simulink model "RelOrbSim"  (R2021b)
settings: Solver=ode3  StartTime=0.0  StopTime=600  FixedStep=1  MaxStep=0.1  RelTol=1e-13  AbsTol=1e-16
values from neighbouring files (symbols this model uses):
  ctrl_flag = 1    [MAIN.m]    (also in MAIN_TestCampaign_1.m)
  g0 = 9.81    [MAIN.m]    (also in MAIN_TestCampaign_1.m)
  Isp = 450    [MAIN.m]    (also in MAIN_TestCampaign_1.m)
  J2_flag = 0    [MAIN.m]    (also in MAIN_TestCampaign_1.m)
  M0 = 12    [MAIN.m]    (also in MAIN_TestCampaign_1.m)
  Mp = 0.5    [MAIN.m]    (also in MAIN_TestCampaign_1.m)
  Y0_Chaser = [7106.14, 0.501, deg2rad(98.31), deg2rad(0), deg2rad(270), deg2rad(0)]'    [MAIN.m]    (also in MAIN_TestCampaign_1.m = [SMA, (ECC+Del_ECC), deg2rad(INC+Del_INC), eg2rad(RAAN), deg)
  Y0_Target = [7106.14, 0.5, deg2rad(98.3), deg2rad(0), deg2rad(270), deg2rad(0)]'    [MAIN.m]    (also in MAIN_TestCampaign_1.m = [SMA, ECC, deg2rad(INC), deg2rad(RAAN), deg2rad(OMEGA), THET)
settings Model: Creator=vvh19  LastModifiedBy=vvh19
settings SolverCC: ZeroCrossAlgorithm=Adaptive
settings DebuggingCC: IgnoredZcDiagnostic=none

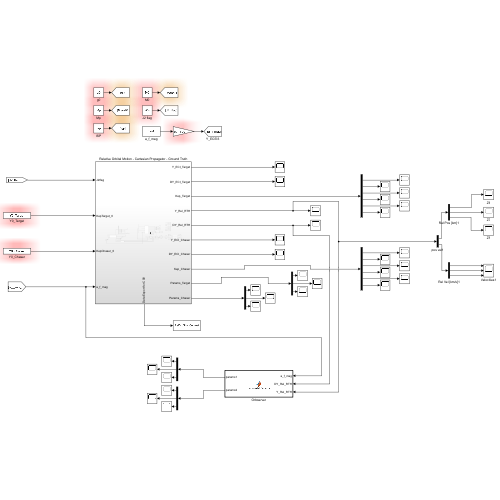
[thumbnail: Simulink's stored preview of the top-level diagram]
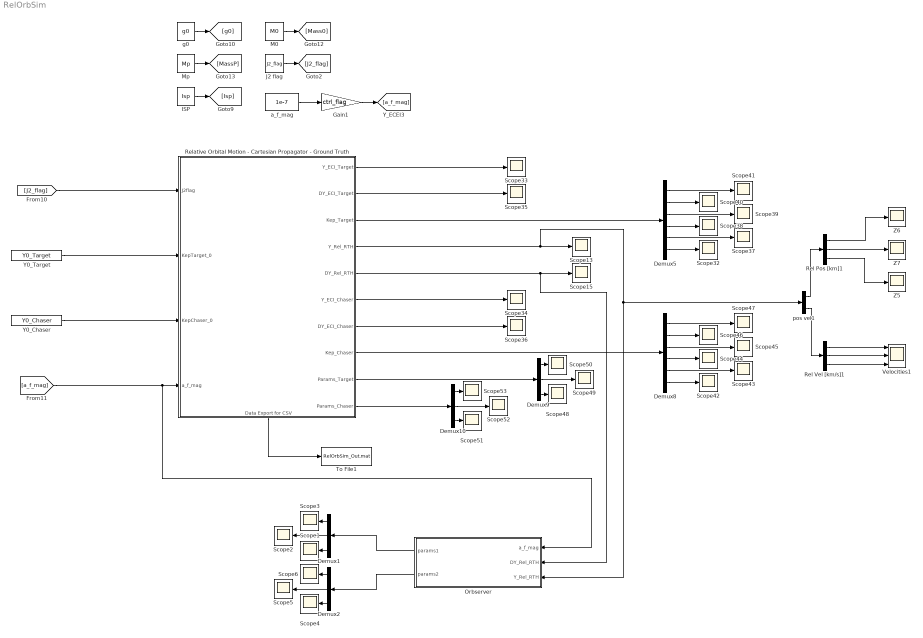
== system RelOrbSim ==
  Demux{1..2,9..10} (4 alike) : Demux  Outputs=3
  Demux5 : Demux  Outputs=6
  Demux8 : Demux  Outputs=6
  Gain1 : Gain  Gain=ctrl_flag
  ISP : Constant  Value=Isp
  J2 flag : Constant  Value=J2_flag
  M0 : Constant  Value=M0
  Mp : Constant  Value=Mp
  Orbserver : MATLAB Function  TreatAsAtomicUnit=on
  Rel Pos [km]1 : Demux  Outputs=3
  Rel Vel [km/s]1 : Demux  Outputs=3
  Relative Orbital Motion - Cartesian Propagator - Ground Truth : Subsystem
      settings: PortSchema="{\"entries\":[{\"content\":{\"sides\":[{\"content\":{\"connectorIds\":[\"In1\",\"In2\",\"In3\",\"In4\"]},\"type\":\"ConnectorPlacement.EquallySpacedRectSide\",\"uuid\":\"460fd9d6-cd5d-4b76-b443-bcd8299910b0\"},{\"content\":{\"connectorIds\":[\"Out1\",\"Out2\",\"Out3\",\"Out4\",\"Out5\",\"Out6\",\"Out7\",\"Out8\",\"Out9\",\"Out10\"],\"side\":\"RIGHT\"},\"type\":\"ConnectorPlacement.EquallySpacedRectSide\",\"uuid\":\"3d6e3c75-f9f1-4d35-a2af-329ac414795a\"},{\"content\":{\"connectorIds\":[],\"side\":\"TOP\"},\"type\":\"ConnectorPlacement.EquallySpacedRectSide\",\"uuid\":\"ebced619-41c7-4fff-b50c-f89432cfa79e\"},{\"content\":{\"connectorIds\":[\"Out11\"],\"side\":\"BOTTOM\"},\"type\":\"ConnectorPlacement.EquallySpacedRectSide\",\"uuid\":\"f646bff0-d8f7-4748-8894-8aba1f3e2913\"}]},\"type\":\"ConnectorPlacement.EquallySpacedConnector\",\"uuid\":\"aa7fbb89-a653-4056-80bd-de050f54cf23\"}],\"packageUris\":[\"http://schema.mathworks.com/mf0/Connector/R2020b\"],\"version\":\"1.0\"}"
  Scope{1..6,13,15,32..53} (30 alike) : Scope
  To File1 : ToFile  Filename=RelOrbSim_Out.mat  MatrixName=Data
  Velocities1 : Scope  NumInputPorts=3
  Y0_Chaser : Constant  Value=Y0_Chaser
  Y0_Target : Constant  Value=Y0_Target
  Z5 : Scope
  Z6 : Scope
  Z7 : Scope
  a_f_mag : Constant  Value=1e-7
  g0 : Constant  Value=g0
  pos vel1 : Demux  Outputs=2
  wires:
  ISP/1 -> [Isp]
  J2 flag/1 -> [J2_flag]
  Mp/1 -> [MassP]
  M0/1 -> [Mass0]
  g0/1 -> [g0]
  Y0_Target/1 -> Relative Orbital Motion - Cartesian Propagator - Ground Truth/2(KepTarget_0)
  Y0_Chaser/1 -> Relative Orbital Motion - Cartesian Propagator - Ground Truth/3(KepChaser_0)
  [J2_flag] -> Relative Orbital Motion - Cartesian Propagator - Ground Truth/1(J2flag)
  Relative Orbital Motion - Cartesian Propagator - Ground Truth/4(Y_Rel_RTH) -> Scope13/1, Orbserver/3(Y_Rel_RTH), pos vel1/1
  Relative Orbital Motion - Cartesian Propagator - Ground Truth/5(DY_Rel_RTH) -> Scope15/1, Orbserver/2(DY_Rel_RTH)
  Relative Orbital Motion - Cartesian Propagator - Ground Truth/1(Y_ECI_Target) -> Scope33/1
  Relative Orbital Motion - Cartesian Propagator - Ground Truth/6(Y_ECI_Chaser) -> Scope34/1
  Relative Orbital Motion - Cartesian Propagator - Ground Truth/2(DY_ECI_Target) -> Scope35/1
  Relative Orbital Motion - Cartesian Propagator - Ground Truth/7(DY_ECI_Chaser) -> Scope36/1
  [a_f_mag] -> Orbserver/1(a_f_mag), Relative Orbital Motion - Cartesian Propagator - Ground Truth/4(a_f_mag)
  Demux5/3 -> Scope39/1
  Demux5/2 -> Scope40/1
  Relative Orbital Motion - Cartesian Propagator - Ground Truth/3(Kep_Target) -> Demux5/1
  Demux5/4 -> Scope38/1
  Demux5/6 -> Scope32/1
  Demux5/1 -> Scope41/1
  Demux5/5 -> Scope37/1
  Demux8/5 -> Scope43/1
  Demux8/1 -> Scope47/1
  Demux8/6 -> Scope42/1
  Demux8/4 -> Scope44/1
  Relative Orbital Motion - Cartesian Propagator - Ground Truth/8(Kep_Chaser) -> Demux8/1
  Demux8/2 -> Scope46/1
  Demux8/3 -> Scope45/1
  Relative Orbital Motion - Cartesian Propagator - Ground Truth/11(Data Export for CSV) -> To File1/1
  Demux9/2 -> Scope49/1
  Demux9/3 -> Scope48/1
  Demux9/1 -> Scope50/1
  Relative Orbital Motion - Cartesian Propagator - Ground Truth/9(Params_Target) -> Demux9/1
  Demux10/1 -> Scope53/1
  Demux10/3 -> Scope51/1
  Demux10/2 -> Scope52/1
  Relative Orbital Motion - Cartesian Propagator - Ground Truth/10(Params_Chaser) -> Demux10/1
  pos vel1/1 -> Rel Pos [km]1/1
  Rel Pos [km]1/1 -> Z6/1
  Rel Pos [km]1/3 -> Z5/1
  pos vel1/2 -> Rel Vel [km/s]1/1
  Rel Pos [km]1/2 -> Z7/1
  Rel Vel [km/s]1/1 -> Velocities1/1
  Rel Vel [km/s]1/2 -> Velocities1/2
  Rel Vel [km/s]1/3 -> Velocities1/3
  Gain1/1 -> [a_f_mag]
  a_f_mag/1 -> Gain1/1
  Demux1/1 -> Scope3/1
  Demux1/3 -> Scope1/1
  Orbserver/1(params1) -> Demux1/1
  Demux1/2 -> Scope2/1
  Demux2/2 -> Scope5/1
  Demux2/3 -> Scope4/1
  Demux2/1 -> Scope6/1
  Orbserver/2(params2) -> Demux2/1

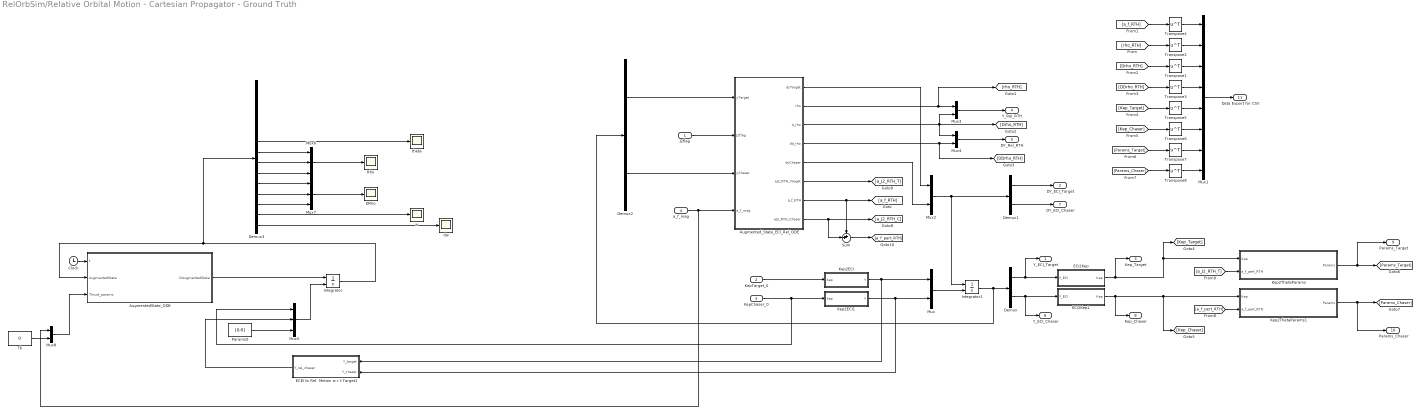
== system RelOrbSim/Relative Orbital Motion - Cartesian Propagator - Ground Truth ==
  J2flag : Inport
  KepTarget_0 : Inport  Port=2
  KepChaser_0 : Inport  Port=3
  a_f_mag : Inport  Port=4
  AugmentedState_ODE : MATLAB Function  TreatAsAtomicUnit=on
  Augmented_State_ECI_Rel_ODE : MATLAB Function  TreatAsAtomicUnit=on
  Clock : Clock
  DRho : Scope
  Demux : Demux  Outputs=2
  Demux1 : Demux  Outputs=2
  Demux2 : Demux  Outputs=2
  Demux3 : Demux  Outputs=14
  ECEI to Rel. Motion w.r.t Target1 : MATLAB Function  TreatAsAtomicUnit=on
  ECI2Kep : MATLAB Function  TreatAsAtomicUnit=on
  ECI2Kep1 : MATLAB Function  TreatAsAtomicUnit=on
  Integrator : Integrator  InitialConditionSource=external
  Integrator1 : Integrator  InitialConditionSource=external  AbsoluteTolerance=1e-14
  Kep2ECI : MATLAB Function  TreatAsAtomicUnit=on
  Kep2ECI1 : MATLAB Function  TreatAsAtomicUnit=on
  Kep2ThetaParams : MATLAB Function  TreatAsAtomicUnit=on
  Kep2ThetaParams1 : MATLAB Function  TreatAsAtomicUnit=on
  Mux{,2..4,8} (5 alike) : Mux  Inputs=2
  Mux1 : Mux  Inputs=8
  Mux5 : Mux  Inputs=3
  Mux6 : Mux  Inputs=3
  Mux7 : Mux  Inputs=3
  Params0 : Constant  Value=[0;0]
  Rho : Scope
  Sum : Sum  Inputs=++|
  Tb : Constant  Value=0
  Transpose{1..8} (8 alike) : Math  Operator=transpose  SaturateOnIntegerOverflow=on
  dw : Scope
  theta : Scope
  w : Scope
  Y_ECI_Target : Outport
  DY_ECI_Target : Outport  Port=2
  Kep_Target : Outport  Port=3
  Y_Rel_RTH : Outport  Port=4
  DY_Rel_RTH : Outport  Port=5
  Y_ECI_Chaser : Outport  Port=6
  DY_ECI_Chaser : Outport  Port=7
  Kep_Chaser : Outport  Port=8
  Params_Target : Outport  Port=9
  Params_Chaser : Outport  Port=10
  Data Export for CSV : Outport  Port=11
  wires:
  J2flag/1 -> Augmented_State_ECI_Rel_ODE/2(J2flag)
  Mux/1 -> Integrator1/2
  KepChaser_0/1 -> Mux5/1, Kep2ECI1/1(kep)
  KepTarget_0/1 -> Kep2ECI/1(kep)
  Kep2ECI/1(Y) -> Mux/1, ECEI to Rel. Motion w.r.t Target1/1(Y_target)
  Kep2ECI1/1(Y) -> ECEI to Rel. Motion w.r.t Target1/2(Y_chaser), Mux/2
  Integrator1/1 -> Demux2/1, Demux/1
  Demux/1 -> ECI2Kep/1(Y_ECI), Y_ECI_Target/1
  Demux/2 -> ECI2Kep1/1(Y_ECI), Y_ECI_Chaser/1
  Mux2/1 -> Demux1/1, Integrator1/1
  Augmented_State_ECI_Rel_ODE/1(dyTarget) -> Mux2/1
  Augmented_State_ECI_Rel_ODE/5(dyChaser) -> Mux2/2
  Demux1/2 -> DY_ECI_Chaser/1
  Demux1/1 -> DY_ECI_Target/1
  Demux2/2 -> Augmented_State_ECI_Rel_ODE/3(yChaser)
  Demux2/1 -> Augmented_State_ECI_Rel_ODE/1(yTarget)
  Augmented_State_ECI_Rel_ODE/2(rho) -> [rho_RTH], Mux3/1
  Augmented_State_ECI_Rel_ODE/3(d_rho) -> Mux3/2, [Drho_RTH], Mux4/1
  Augmented_State_ECI_Rel_ODE/4(dd_rho) -> [DDrho_RTH], Mux4/2
  Mux3/1 -> Y_Rel_RTH/1
  Mux4/1 -> DY_Rel_RTH/1
  a_f_mag/1 -> Mux8/1, Augmented_State_ECI_Rel_ODE/4(a_f_mag)
  ECI2Kep/1(Kep) -> [Kep_Target], Kep2ThetaParams/1(Kep), Kep_Target/1
  ECI2Kep1/1(Kep) -> Kep2ThetaParams1/1(Kep), [Kep_Chaser], Kep_Chaser/1
  [DDrho_RTH] -> Transpose3/1
  [Drho_RTH] -> Transpose1/1
  [rho_RTH] -> Transpose2/1
  [a_f_RTH] -> Transpose4/1
  [Kep_Target] -> Transpose5/1
  [Kep_Chaser] -> Transpose6/1
  Transpose4/1 -> Mux1/1
  Transpose2/1 -> Mux1/2
  Transpose1/1 -> Mux1/3
  Transpose3/1 -> Mux1/4
  Transpose5/1 -> Mux1/5
  Transpose6/1 -> Mux1/6
  Mux1/1 -> Data Export for CSV/1
  Kep2ThetaParams/1(Params) -> [Params_Target], Params_Target/1
  Kep2ThetaParams1/1(Params) -> Params_Chaser/1, [Params_Chaser]
  [Params_Chaser] -> Transpose8/1
  [Params_Target] -> Transpose7/1
  Transpose7/1 -> Mux1/7
  Transpose8/1 -> Mux1/8
  Augmented_State_ECI_Rel_ODE/7(a_f_RTH) -> Sum/1, [a_f_RTH]
  Augmented_State_ECI_Rel_ODE/8(aJ2_RTH_Chaser) -> Sum/2, [a_J2_RTH_C]
  Augmented_State_ECI_Rel_ODE/6(aJ2_RTH_Target) -> [a_J2_RTH_T]
  Sum/1 -> [a_f_pert_RTH]
  [a_f_pert_RTH] -> Kep2ThetaParams1/2(a_f_pert_RTH)
  [a_J2_RTH_T] -> Kep2ThetaParams/2(a_f_pert_RTH)
  AugmentedState_ODE/1(DAugmentedState) -> Integrator/1
  Clock/1 -> AugmentedState_ODE/1(t)
  Integrator/1 -> Demux3/1, AugmentedState_ODE/2(AugmentedState)
  Mux5/1 -> Integrator/2
  ECEI to Rel. Motion w.r.t Target1/1(Y_rel_chaser) -> Mux5/2
  Params0/1 -> Mux5/3
  Demux3/7 -> Mux6/1
  Demux3/8 -> Mux6/2
  Demux3/9 -> Mux6/3
  Demux3/10 -> Mux7/1
  Demux3/11 -> Mux7/2
  Demux3/12 -> Mux7/3
  Mux6/1 -> Rho/1
  Mux7/1 -> DRho/1
  Demux3/13 -> w/1
  Demux3/14 -> dw/1
  Demux3/6 -> theta/1
  Tb/1 -> Mux8/2
  Mux8/1 -> AugmentedState_ODE/3(Thrust_params)

== matlab function RelOrbSim/Relative Orbital Motion - Cartesian Propagator - Ground Truth/AugmentedState_ODE ==
  data: DAugmentedState output size=14,1; t input; AugmentedState input; Thrust_params input
function DAugmentedState = AugmentedState_ODE( t, AugmentedState, Thrust_params )
% AugmentedState = [Kep; Rel; Params];
% DParams are computed independantly of Params
% Hence input values of Params need not be accurate

% Thrust_params = [T0; Tb];

%%%%%%%%%%%%%%%%%%%%%%%%%%%%%%%%%%%%%%%%%%%%%%%%%%%%%%%%%%%%%%%%%%%%%%%%%%%
mu = 3.24858599E+5; % From DE405
J2 = 0.1082626925638815e-2; % Definition in Wertz, SMAD
R_E = 6378.1363; % To be used for J2 value compatibility
% Assuming Exponential Thrust Profile --> T = T0 * e^(-b*t);

T0 = Thrust_params(1);       Tb = Thrust_params(2);
a_f_mag = T0 * exp(-Tb*t);
%%%%%%%%%%%%%%%%%%%%%%%%%%%%%%%%%%%%%%%%%%%%%%%%%%%%%%%%%%%%%%%%%%%%%%%%%%%
a = AugmentedState(1);   e = AugmentedState(2);   i = AugmentedState(3);
OM = AugmentedState(4);  om = AugmentedState(5);  theta = AugmentedState(6);
X = AugmentedState(7);   Y = AugmentedState(8);   Z = AugmentedState(9); 
VX = AugmentedState(10); VY = AugmentedState(11); VZ = AugmentedState(12); 
%%%%%%%%%%%%%%%%%%%%%%%%%%%%%%%%%%%%%%%%%%%%%%%%%%%%%%%%%%%%%%%%%%%%%%%%%%%
Rho_cap = ([X;Y;Z]/norm([X;Y;Z]));
DRho_cap = ([VX;VY;VZ]/norm([VX;VY;VZ]));
DDRho_cap = Rho_cap*1e-6; % Temporary and also very negligible value (I Think)
a_f_RTH = -(Rho_cap*a_f_mag);
Da_f_RTH = -(Rho_cap*a_f_mag*(-Tb) + a_f_mag*DRho_cap);
DDa_f_RTH = -(Rho_cap*a_f_mag*Tb^2 + 2*a_f_mag*(-Tb)*DRho_cap + a_f_mag*DDRho_cap);

p = a * ( 1 - e^2 );
h = sqrt( p * mu );
r = p / ( 1 + e * cos( theta ) );

aJ2_vect_RTH = -3/2 * J2 * mu * R_E.^2 / r.^4 * ...
    [ 1 - 3 * sin(i).^2 * sin( theta + om ).^2; ...
    sin(i).^2 * sin( 2 * (theta + om) ); ...
    sin( 2 * i ) * sin( theta + om ) ];

% Neglecting Derivatives of a_J2_RTH in derivatives of external RTH acceleration
% To be included later
DaJ2_vect_RTH = [0;0;0];    DDaJ2_vect_RTH = [0;0;0];

a_tot_RTH = a_f_RTH + aJ2_vect_RTH;
Da_tot_RTH = Da_f_RTH + DaJ2_vect_RTH;
DDa_tot_RTH = DDa_f_RTH + DDaJ2_vect_RTH;

a_r = a_tot_RTH(1);         a_t = a_tot_RTH(2);         a_h = a_tot_RTH(3);
Da_r = Da_tot_RTH(1);       Da_t = Da_tot_RTH(2);       Da_h = Da_tot_RTH(3);
DDa_r = DDa_tot_RTH(1);     DDa_t = DDa_tot_RTH(2);     DDa_h = DDa_tot_RTH(3);
%%%%%%%%%%%%%%%%%%%%%%%%%%%%%%%%%%%%%%%%%%%%%%%%%%%%%%%%%%%%%%%%%%%%%%%%%%%
Da = 2 * a.^2 / h * ( e * sin( theta ) * a_r + p / r * a_t );
De = 1 / h * ( p * sin( theta ) * a_r + ( ( p + r ) * cos( theta ) + r * e ) * a_t ); 
Di = r * cos( theta + om ) / h * a_h;
DOM = r * sin( theta + om ) / ( h * sin(i) ) * a_h;
Dom = 1 / ( h * e ) * ( -p * cos( theta ) * a_r + ( p + r ) * sin( theta ) * a_t ) - r * sin( theta + om ) * cos( i ) / ( h * sin(i) ) * a_h;
%%%%%%%%%%%%%%%%%%%%%%%%%%%%%%%%%%%%%%%%%%%%%%%%%%%%%%%%%%%%%%%%%%%%%%%%%%%
Dtheta = h / r.^2 + 1 / ( e * h ) * (p * cos( theta ) * a_r - ( p + r ) * sin( theta ) * a_t ); 

Dr = e * p * Dtheta * sin( theta ) / ( 1 + e * cos ( theta ) )^2;
DDtheta = (-2*h*Dr/r^3) + (1/e/h)*(p*Da_r*cos(theta) - a_r*Dtheta*sin(theta))...
    - (1/e/h)*(Da_t*sin(theta)*(p+r) + a_t*Dtheta*cos(theta)*(p+r) + a_t*sin(theta)*Dr);

DDr = e*p*(2*DDtheta*sin(theta)*(1+e*cos(theta)) + Dtheta^2*( 2*cos(theta) - e*(cos(2*theta) - 3) ) ) / (2*(1+e*cos(theta))^3);
DDDtheta = ((6*h*Dr^2 - 2*h*r*DDr)/r^4) - (1/e/h)*( p*(-DDa_r*cos(theta) + 2*Da_r*Dtheta*sin(theta) + a_r*(DDtheta*sin(theta) + Dtheta^2*cos(theta)) ) )...
    - (1/e/h)*(2*Dtheta*cos(theta)*(Da_t*(p+r) + a_t*Dr) + sin(theta)*(DDa_t*(p+r) + 2*Da_r*Dr + a_r*DDr) + a_t*(p+r)*(DDtheta*cos(theta) - Dtheta^2*sin(theta)));
%%%%%%%%%%%%%%%%%%%%%%%%%%%%%%%%%%%%%%%%%%%%%%%%%%%%%%%%%%%%%%%%%%%%%%%%%%%
kw3_2 = mu/r^3;     w = Dtheta;         dw = DDtheta;
DX = VX;            DY = VY;            DZ = VZ;
DVX = (2*kw3_2 + w^2)*X + dw*Y + 2*w*VY + a_r;
DVY = -dw*X + (w^2 - kw3_2)*Y - 2*w*VX + a_t;
DVZ = -(kw3_2)*Z + a_h;
%%%%%%%%%%%%%%%%%%%%%%%%%%%%%%%%%%%%%%%%%%%%%%%%%%%%%%%%%%%%%%%%%%%%%%%%%%%
DKep = [Da;De;Di;DOM;Dom;Dtheta];
DRel = [DX;DY;DZ;DVX;DVY;DVZ];
DParams = [DDtheta; DDDtheta];

DAugmentedState = [DKep; DRel; DParams];
end

== matlab function RelOrbSim/Relative Orbital Motion - Cartesian Propagator - Ground Truth/ECEI to Rel. Motion w.r.t Target1 ==
  data: Y_target input; Y_rel_chaser output; Y_chaser input
function Y_rel_chaser = ECEI2Hill( Y_target, Y_chaser)

% Initialisation
r_t = Y_target(1:3);    v_t = Y_target(4:6);
r_c = Y_chaser(1:3);    v_c = Y_chaser(4:6);

% Construct Target Centered LVLH Frame
x_cap = r_t./norm(r_t);
z_cap = ( cross(r_t, v_t) ./ norm(cross(r_t, v_t)) );
y_cap = cross(z_cap, x_cap) ./ norm(cross(z_cap, x_cap));

T = [x_cap, y_cap, z_cap]';

%
rho_ECI = r_c - r_t;
rho_dot_ECI = v_c - v_t;

rho = T*rho_ECI;
rho_dot = T*rho_dot_ECI;

% Construct Rel. State Vector of Chaser in target's LVLH Frame
Y_rel_chaser = [rho; rho_dot];

end

== matlab function RelOrbSim/Orbserver ==
  data: a_f_mag input; DY_Rel_RTH input; Y_Rel_RTH input; params1 output; params2 output
function [params1, params2] = EstimateParams(a_f_mag, DY_Rel_RTH, Y_Rel_RTH)

rho = Y_Rel_RTH(1:3);  Drho = Y_Rel_RTH(4:6);  DDrho = DY_Rel_RTH(4:6);

rho_cap_RTH = rho./norm(rho);
thrust_cap_RTH = -rho_cap_RTH; 
a_f_RTH = thrust_cap_RTH*a_f_mag;

gamma = (DDrho(3) - a_f_RTH(3))/rho(3);

A = DDrho(1) + 2*gamma*rho(1) - a_f_RTH(1);
B = DDrho(2) - gamma*rho(2) - a_f_RTH(2);

C1 = (2*rho(1)*Drho(2) - 2*rho(2)*Drho(1));
C2 = (rho(1)^2 + rho(2)^2);
C3 = (B*rho(2) + A*rho(1));

square_root = sqrt( complex(C1^2 + 4*C2*C3) );

w1 = real(-C1 + square_root)/(2*C2);
w2 = real(-C1 - square_root)/(2*C2);

Dw1 = (w1*(w1*rho(2) - 2*Drho(2)) - B)/rho(1);
Dw2 = (w2*(w2*rho(2) - 2*Drho(2)) - B)/rho(1);

kw3_2 = -gamma;

params1 = [kw3_2; Dw1; w1];
params2 = [kw3_2; Dw2; w2];

end

== matlab function RelOrbSim/Relative Orbital Motion - Cartesian Propagator - Ground Truth/Augmented_State_ECI_Rel_ODE ==
  data: dyTarget output size=6,1; rho output size=3,1; d_rho output size=3,1; dd_rho output size=3,1; yTarget input; J2flag input; yChaser input; dyChaser output size=6,1; aJ2_RTH_Target output size=3,1; a_f_mag input; a_f_RTH output size=3,1; aJ2_RTH_Chaser output size=3,1
function [dyTarget, rho, d_rho, dd_rho, dyChaser, aJ2_RTH_Target, a_f_RTH, aJ2_RTH_Chaser] = ode_2BP_Earth(yTarget, J2flag, yChaser, a_f_mag)

mu = 3.98600433e+5; % From DE405
R_E = 6378.1363; % use for J2 only [km] 

if J2flag == 0
    J2 = 0;
else  
    J2 = 0.1082626925638815e-2; % J2 value (Definition in Wertz, SMAD)
end

% Relative RTH State Vector
r_T = yTarget(1:3);    v_T = yTarget(4:6);     
r_C = yChaser(1:3);    v_C = yChaser(4:6);      

% Construct Target Centered RTH Frame
x_cap = r_T./norm(r_T);
z_cap = ( cross(r_T, v_T) ./ norm(cross(r_T, v_T)) );
y_cap = cross(z_cap, x_cap) ./ norm(cross(z_cap, x_cap));
T = [x_cap, y_cap, z_cap]';

rho_ECI = r_C - r_T;    rho_dot_ECI = v_C - v_T;    

% Control Accelerations
rho_cap_ECI = rho_ECI./norm(rho_ECI);
thrust_cap_ECI = -rho_cap_ECI;
a_f_ECI = thrust_cap_ECI*a_f_mag;

% Outputs - 1
[dyTarget, aJ2_vect_ECEI_Target] = ode_2BP_perturbed_J2(yTarget, mu, R_E, J2, [0;0;0] );
[dyChaser, aJ2_vect_ECEI_Chaser] = ode_2BP_perturbed_J2(yChaser, mu, R_E, J2, a_f_ECI );

dv_T = dyTarget(4:6);      dv_C = dyChaser(4:6);       rho_dotdot_ECI = dv_C - dv_T;

% Outputs - 2
rho = T*rho_ECI;        d_rho = T*rho_dot_ECI;    dd_rho =  T*rho_dotdot_ECI;
aJ2_RTH_Target = T*aJ2_vect_ECEI_Target;    aJ2_RTH_Chaser = T*aJ2_vect_ECEI_Chaser;

rho_cap_RTH = rho./norm(rho);
thrust_cap_RTH = -rho_cap_RTH; 
a_f_RTH = thrust_cap_RTH*a_f_mag;

end

%%%%%%%%%%%%%%%%%%%%%%%%%%%%%%%%%%%%%%%%%%%%%%%%%%%%%%%%%%%%%%%%%%%%%%%%%%%

function [dy, aJ2_vect_ECEI] = ode_2BP_perturbed_J2(y, mu, R_E, J2, a_f_ECI )
r = y(1:3);
r_norm = norm(r);
v = y(4:6);

aJ2_vect_ECEI = 3/2 * J2 * mu * R_E^2 / r_norm^5 *       ... % Multiplicative constant
    [ r(1) * ( 5 * (r(3) / r_norm)^2 - 1 );   ... % x-component
      r(2) * ( 5 * (r(3) / r_norm)^2 - 1 );   ... % y-component
      r(3) * ( 5 * (r(3) / r_norm)^2 - 3 )];      % z-component

dy = [ v; -mu ./ r_norm.^3 .* r + aJ2_vect_ECEI + a_f_ECI];

end

== matlab function RelOrbSim/Relative Orbital Motion - Cartesian Propagator - Ground Truth/Kep2ECI ==
  data: Y output; kep input
function Y = Kep2Car( kep )
%% Inputs
a = kep(1);     e = kep(2);     i = kep(3);
OM = kep(4);    om = kep(5);    theta = kep(6);
mu = 3.98600433e+5; % From DE405

%% Calculate r, v in perifocal frame
unit_r = [cos(theta); sin(theta); 0];
unit_theta = [-sin(theta); cos(theta); 0];
P = a.*(1-e.^2);

r_pf = a .* (1 - e.^2) ./ (1 + e .* cos(theta)) * unit_r; % r in perifocal plane
v_r = sqrt( mu ./ P ) .* e .* sin(theta) * unit_r;
v_theta = sqrt( mu ./ P ) .* ( 1 + e .* cos(theta) ) * unit_theta;

v_pf = v_r + v_theta;

%% Calculate rotation matrix

R_OM  = [  cos(OM), sin(OM), 0       ;
          -sin(OM), cos(OM), 0       ;
           0,       0,       1      ];

R_i  = [   1,       0,       0       ;
           0,       cos(i),  sin(i)  ;
           0,      -sin(i),  cos(i) ];

R_om = [   cos(om), sin(om), 0                     
          -sin(om), cos(om), 0
           0,       0,       1,     ];

R_ECEI2PF = R_om*R_i*R_OM;

r = R_ECEI2PF'*r_pf;
v = R_ECEI2PF'*v_pf;

%% Generate State Vector
Y = [r;v];
end

== matlab function RelOrbSim/Relative Orbital Motion - Cartesian Propagator - Ground Truth/Kep2ThetaParams1 ==
  data: Params output size=3,1; Kep input; a_f_pert_RTH input
function Params = Kep2ThetaParams(Kep, a_f_pert_RTH)
%% Inputs
a = Kep(1);     e = Kep(2);     theta = Kep(6);
a_r = a_f_pert_RTH(1);      a_t = a_f_pert_RTH(2);      a_h = a_f_pert_RTH(3);

mu = 3.98600433e+5; % From DE405

r = a*(1-e^2)/(1+e*cos(theta));

kw3_2 = mu/r^3;
% dw = -2*mu*e*sin(theta) / r^3;
% w = sqrt( mu * a*(1-e^2) ) / r^2;
% 
% Params = [kw3_2; dw; w];

% Trial - Also find derivative of "w" in presence of perturbations
h = sqrt( mu * a*(1-e^2) );
p = a*(1-e^2);

w =  h / r.^2 + 1 / ( e * h ) * (p * cos( theta ) * a_r - ( p + r ) * sin( theta ) * a_t );

r_dot = e * p * w * sin( theta ) / ( 1 + e * cos( theta ) )^2;

dw = ( -2 * h * r_dot / r^3 ) + ( 1 / ( e * h ) ) *...
    ( ( w * -( a_r * p * sin(theta) + a_t * r * cos(theta) + a_t * p * cos(theta) ) )...
        - a_t * sin(theta) * r_dot );

Params = [kw3_2; dw; w];

end

== matlab function RelOrbSim/Relative Orbital Motion - Cartesian Propagator - Ground Truth/Kep2ECI1 ==
  data: Y output; kep input
function Y = Kep2Car( kep )
%% Inputs
a = kep(1);     e = kep(2);     i = kep(3);
OM = kep(4);    om = kep(5);    theta = kep(6);
mu = 3.98600433e+5; % From DE405

%% Calculate r, v in perifocal frame
unit_r = [cos(theta); sin(theta); 0];
unit_theta = [-sin(theta); cos(theta); 0];
P = a.*(1-e.^2);

r_pf = a .* (1 - e.^2) ./ (1 + e .* cos(theta)) * unit_r; % r in perifocal plane
v_r = sqrt( mu ./ P ) .* e .* sin(theta) * unit_r;
v_theta = sqrt( mu ./ P ) .* ( 1 + e .* cos(theta) ) * unit_theta;

v_pf = v_r + v_theta;

%% Calculate rotation matrix

R_OM  = [  cos(OM), sin(OM), 0       ;
          -sin(OM), cos(OM), 0       ;
           0,       0,       1      ];

R_i  = [   1,       0,       0       ;
           0,       cos(i),  sin(i)  ;
           0,      -sin(i),  cos(i) ];

R_om = [   cos(om), sin(om), 0                     
          -sin(om), cos(om), 0
           0,       0,       1,     ];

R_ECEI2PF = R_om*R_i*R_OM;

r = R_ECEI2PF'*r_pf;
v = R_ECEI2PF'*v_pf;

%% Generate State Vector
Y = [r;v];
end

== matlab function RelOrbSim/Relative Orbital Motion - Cartesian Propagator - Ground Truth/ECI2Kep ==
  data: Kep output size=6,1; Y_ECI input
function Kep = Car2Kep(Y_ECI)
% Calculate parameters
r_ECI = Y_ECI(1:3);
v_ECI = Y_ECI(4:6);
mu = 3.98600433e+5; % From DE405

% This tolerance is required to have accurate results from MATLAB
tol = .2e-15;

% Define xyz axis
x = [ 1, 0, 0 ];
y = [ 0, 1, 0 ];
z = [ 0, 0, 1 ];

r_norm = norm(r_ECI);

% Calculate semi-major axis
a = 1 ./ ( 2 ./ r_norm - norm(v_ECI).^2 ./ mu );

% Calculate angular momentum vector
h_ECI = cross( r_ECI, v_ECI );

% Calculate eccentricity vector
e = cross( v_ECI, h_ECI ) ./ mu - r_ECI ./ r_norm;
e_norm = norm(e);

% Calculate inclination
i = acos( dot( h_ECI, z ) ./ norm(h_ECI) ); % 0<i<pi
%%%%%%%%%%%%%%%%%%%%%%%%%%%%%%%%%%%%%%%%%%%%%%%%%%%%%%%%%%%%%%%%%%%%%%%%%%%
if i - tol < 0
    % RAAN is undefined if i = 0 ( i < tol )
    OM = 0;
    AN = [1;0;0];
else
    % RAAN is defined
    % Calculate ascending node (AN)
    AN = cross( z, h_ECI ) ./ norm( cross( z, h_ECI ) ); % Ascending node unit vector
    % Solve OM angle ambiguity
    if dot( AN, y ) > 0 % 0<OM<2pi
        OM = acos( dot( x, AN ) );
    elseif dot( AN, y ) < 0 % 0<OM<2pi
        OM = 2*pi - acos( dot( x, AN ) );
    else % dot( AN, y ) = 0
        % In this case, OM could be 0 or 180 ???? -> Check if it can
        % actually be 180 because idk
        OM = 0;
    end
end

if e_norm - tol > 0
    % om is defined
    % Solve om angular ambiguity
    if dot( z, e ) >= 0
        om = acos( dot(AN, e) ./ e_norm );
    elseif dot( z, e ) < 0
        om = 2*pi - acos( dot(AN, e) ./ e_norm );
    else
        om = 0;
    end
else
    % om is undefined if e = 0 ( e < tol )
    om = 0;
end

if e_norm - tol > 0
    % theta can be calculated from eccentricity vector if e_norm > tol
    % Solve theta angular ambiguity
    K = dot( r_ECI, e ) ./ ( r_norm .* e_norm );
    k = max(min(K,1),-1);
    if dot( r_ECI, v_ECI ) >= 0
        theta = acos( k );
    elseif dot( r_ECI, v_ECI ) < 0
        theta = 2*pi - acos( k );
    else
        theta = 0;
    end
else
    % theta cannot be calculated from eccentricity vector if e_norm < tol
    % Set theta to start from x-axis and solve for angular ambiguity
    if dot( r_ECI, v_ECI ) >= 0
        theta = acos( dot( r_ECI, x ) ./ ( r_norm ) );
    elseif dot( r_ECI, v_ECI ) < 0
        theta = 2*pi - acos( dot( r_ECI, x ) ./ ( r_norm ) );
    else
        theta = 0;
    end
    % If you arrive in this if, e_norm < tol -> it was actually 0
    e_norm = 0;
end
%%%%%%%%%%%%%%%%%%%%%%%%%%%%%%%%%%%%%%%%%%%%%%%%%%%%%%%%%%%%%%%%%%%%%%%%%%%
om = om(1);
Kep = zeros(6,1);
Kep = [ a, e_norm, i, OM, om, theta ]';
end

== matlab function RelOrbSim/Relative Orbital Motion - Cartesian Propagator - Ground Truth/ECI2Kep1 ==
  data: Kep output size=6,1; Y_ECI input
function Kep = Car2Kep(Y_ECI)
% Calculate parameters
r_ECI = Y_ECI(1:3);
v_ECI = Y_ECI(4:6);
mu = 3.98600433e+5; % From DE405

% This tolerance is required to have accurate results from MATLAB
tol = .2e-15;

% Define xyz axis
x = [ 1, 0, 0 ];
y = [ 0, 1, 0 ];
z = [ 0, 0, 1 ];

r_norm = norm(r_ECI);

% Calculate semi-major axis
a = 1 ./ ( 2 ./ r_norm - norm(v_ECI).^2 ./ mu );

% Calculate angular momentum vector
h_ECI = cross( r_ECI, v_ECI );

% Calculate eccentricity vector
e = cross( v_ECI, h_ECI ) ./ mu - r_ECI ./ r_norm;
e_norm = norm(e);

% Calculate inclination
i = acos( dot( h_ECI, z ) ./ norm(h_ECI) ); % 0<i<pi
%%%%%%%%%%%%%%%%%%%%%%%%%%%%%%%%%%%%%%%%%%%%%%%%%%%%%%%%%%%%%%%%%%%%%%%%%%%
if i - tol < 0
    % RAAN is undefined if i = 0 ( i < tol )
    OM = 0;
    AN = [1;0;0];
else
    % RAAN is defined
    % Calculate ascending node (AN)
    AN = cross( z, h_ECI ) ./ norm( cross( z, h_ECI ) ); % Ascending node unit vector
    % Solve OM angle ambiguity
    if dot( AN, y ) > 0 % 0<OM<2pi
        OM = acos( dot( x, AN ) );
    elseif dot( AN, y ) < 0 % 0<OM<2pi
        OM = 2*pi - acos( dot( x, AN ) );
    else % dot( AN, y ) = 0
        % In this case, OM could be 0 or 180 ???? -> Check if it can
        % actually be 180 because idk
        OM = 0;
    end
end

if e_norm - tol > 0
    % om is defined
    % Solve om angular ambiguity
    if dot( z, e ) >= 0
        om = acos( dot(AN, e) ./ e_norm );
    elseif dot( z, e ) < 0
        om = 2*pi - acos( dot(AN, e) ./ e_norm );
    else
        om = 0;
    end
else
    % om is undefined if e = 0 ( e < tol )
    om = 0;
end

if e_norm - tol > 0
    % theta can be calculated from eccentricity vector if e_norm > tol
    % Solve theta angular ambiguity
    K = dot( r_ECI, e ) ./ ( r_norm .* e_norm );
    k = max(min(K,1),-1);
    if dot( r_ECI, v_ECI ) >= 0
        theta = acos( k );
    elseif dot( r_ECI, v_ECI ) < 0
        theta = 2*pi - acos( k );
    else
        theta = 0;
    end
else
    % theta cannot be calculated from eccentricity vector if e_norm < tol
    % Set theta to start from x-axis and solve for angular ambiguity
    if dot( r_ECI, v_ECI ) >= 0
        theta = acos( dot( r_ECI, x ) ./ ( r_norm ) );
    elseif dot( r_ECI, v_ECI ) < 0
        theta = 2*pi - acos( dot( r_ECI, x ) ./ ( r_norm ) );
    else
        theta = 0;
    end
    % If you arrive in this if, e_norm < tol -> it was actually 0
    e_norm = 0;
end
%%%%%%%%%%%%%%%%%%%%%%%%%%%%%%%%%%%%%%%%%%%%%%%%%%%%%%%%%%%%%%%%%%%%%%%%%%%
om = om(1);
Kep = zeros(6,1);
Kep = [ a, e_norm, i, OM, om, theta ]';
end

== matlab function RelOrbSim/Relative Orbital Motion - Cartesian Propagator - Ground Truth/Kep2ThetaParams ==
  data: Params output size=3,1; Kep input; a_f_pert_RTH input
function Params = Kep2ThetaParams(Kep, a_f_pert_RTH)
%% Inputs
a = Kep(1);     e = Kep(2);     theta = Kep(6);
a_r = a_f_pert_RTH(1);      a_t = a_f_pert_RTH(2);      a_h = a_f_pert_RTH(3);

mu = 3.98600433e+5; % From DE405

r = a*(1-e^2)/(1+e*cos(theta));

kw3_2 = mu/r^3;
% dw = -2*mu*e*sin(theta) / r^3;
% w = sqrt( mu * a*(1-e^2) ) / r^2;
% 
% Params = [kw3_2; dw; w];

% Trial - Also find derivative of "w" in presence of perturbations
h = sqrt( mu * a*(1-e^2) );
p = a*(1-e^2);

w =  h / r.^2 + 1 / ( e * h ) * (p * cos( theta ) * a_r - ( p + r ) * sin( theta ) * a_t );

r_dot = e * p * w * sin( theta ) / ( 1 + e * cos( theta ) )^2;

dw = ( -2 * h * r_dot / r^3 ) + ( 1 / ( e * h ) ) *...
    ( ( w * -( a_r * p * sin(theta) + a_t * r * cos(theta) + a_t * p * cos(theta) ) )...
        - a_t * sin(theta) * r_dot );

Params = [kw3_2; dw; w];

end
